simulink model "window"  (R2020a)
settings: Solver=VariableStepAuto  StartTime=0.0  StopTime=20000/f  RelTol=1e-3
InitFcn:
  | f = 256e6;
  | fs = 1.024e9;
  | delay = 0;
values from neighbouring files (symbols this model uses):
  fc_rx = 110e6    (= 110000000)    [spectrum_analyzer_setup.m]
  fc_tx = 110e6    (= 110000000)    [spectrum_analyzer_setup.m]
  SymbolRate = 1e6    (= 1000000)    [spectrum_analyzer_setup.m]
undefined symbols (not defined in the file or in its folder): designMultirateFIR, F_CICI, F_RRC, firhalfband
libraries: hdlsllib x14, dspmlti4 x6, dspfdesign x4, dspsrcs4 x3, simulink x2, dsparch4 x2, commfilt2 x2, commrandsrc3 x1, commdigbbndpm3 x1
settings Model: SimulationMode=accelerator  Creator=ckb13136  LastModifiedBy=david
settings DataIOCC: ReturnWorkspaceOutputs=off
settings OptimizationCC: BlockReduction=off  ConditionallyExecuteInputs=off  DefaultParameterBehavior=Inlined
settings DebuggingCC: AlgebraicLoopMsg=error  ArithmeticOperatorsInVariantConditions=warning
settings HardwareCC: ProdBitPerPointer=32  ProdBitPerSizeT=32  ProdBitPerPtrDiffT=32  ProdLargestAtomicFloat=None  ProdIntDivRoundTo=Undefined  ProdEndianess=Unspecified  ProdWordSize=32  ProdHWDeviceType=ASIC/FPGA->ASIC/FPGA  TargetBitPerPointer=64  TargetBitPerSizeT=64  TargetBitPerPtrDiffT=64  TargetLongLongMode=on  TargetIntDivRoundTo=Zero  TargetEndianess=LittleEndian  TargetWordSize=64  TargetHWDeviceType=Custom Processor->MATLAB Host Computer  ProdEqTarget=off
settings SFSimCC: SimUseLocalCustomCode=off  CustomCodeUndefinedFunction=UseInterfaceOnly
settings RTWCC: RTWUseLocalCustomCode=off

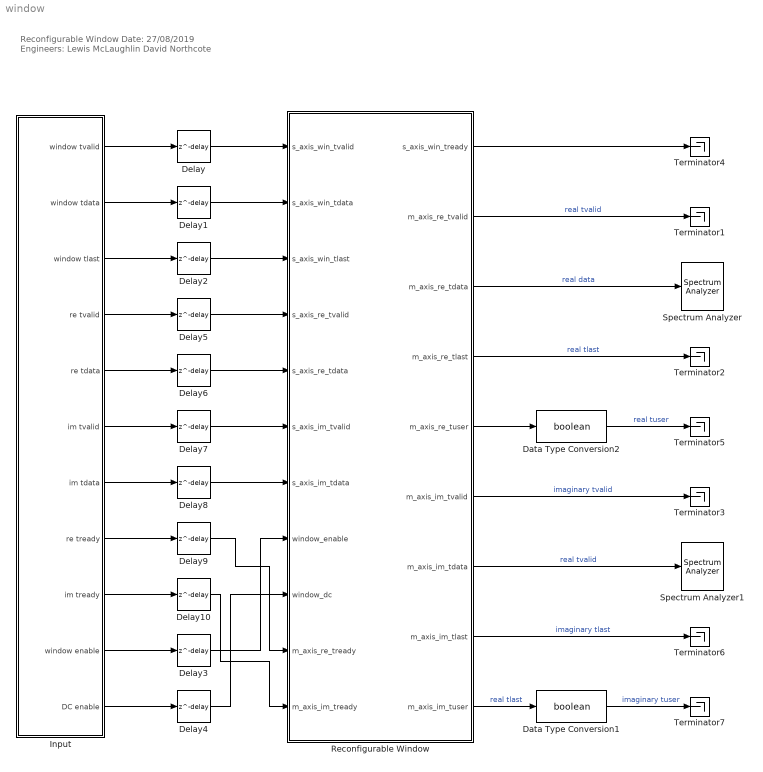
== system window ==
  note: Reconfigurable Window
      | Date: 27/08/2019
      | Engineers: Lewis McLaughlin
      | David Northcote
  Data Type Conversion1 : DataTypeConversion  OutDataTypeStr=boolean
  Data Type Conversion2 : DataTypeConversion  OutDataTypeStr=boolean
  Delay{,1..10} (11 alike) : Delay  DelayLength=delay
  Input : Subsystem  mask{window_length_mask=2048, window_type_mask=Debug, factor=1, f_hz=1e6, typeIn=Constant High, amplitude=0.990, DC=0.0, win_en=on, DC_en=off}
      mask prompts: window_length_mask "Window Length:"; window_type_mask "Window Type:"; factor "Downsample Factor:"; f_hz "Sine Frequency (Hz):"; typeIn "Input Type:"; DC "DC Component"; win_en "Window"; DC_en "DC Block"
      mask init:
      | % Parameters
      | if strcmpi(get_param(gcb, 'window_type_mask'), 'Hamming')
      |     window_type = 0;
      | elseif strcmpi(get_param(gcb, 'window_type_mask'), 'Hann')
      |     window_type = 1;
      | elseif strcmpi(get_param(gcb, 'window_type_mask'), 'Blackman')
      |     window_type = 2;
      | elseif strcmpi(get_param(gcb, 'window_type_mask'), 'Rectangular')
      |     window_type = 3;
      | elseif strcmpi(get_param(gcb, 'window_type_mask'), 'Debug')
      |     window_type = 4;
      | end
      | 
      | window_length = str2num(get_param(gcb, 'window_length_mask'));
      | 
      | % Input
      | if strcmpi(get_param(gcb,'typeIn'),'Constant High')
      |     input_type = 0;
      | elseif strcmpi(get_param(gcb,'typeIn'),'Sine Wave')
      |     input_type = 1;
      | elseif strcmpi(get_param(gcb,'typeIn'),'RF')
      |     input_type = 2;
      | end
      mask TypeOptions window_type_mask: Hamming | Hann | Blackman | Rectangular | Debug
      mask TypeOptions typeIn: Sine Wave | Constant High | RF
      mask DialogControl DescGroupVar Prompt: Input to Window Block
      mask DialogControl DescTextVar Prompt: Update the window parameters and input type as the system runs. A constant high input allows for the window shape to be observed with respect to time.
      mask DialogControl InputGroupVar Prompt: Input
      mask DialogControl EnableGroupVat Prompt: Enable
  Reconfigurable Window : Subsystem  AncestorBlock=lib_window/Reconfigurable Window  TreatAsAtomicUnit=on  VariantControl=Variant  mask{window_size=2048}
      mask prompts: window_size "Maximum Window Length:"
      mask DialogControl DescGroupVar Prompt: AXI-Stream Window
      mask DialogControl DescTextVar Prompt: When changing the window size, ensure the FIFOs under this mask are at least double maximum window size. Window size should be a power of two.
  Spectrum Analyzer : SpectrumAnalyzer
  Spectrum Analyzer1 : SpectrumAnalyzer
  Terminator{1..7} (7 alike) : Terminator
  wires:
  Input/4(re tvalid) -> Delay5/1
  Input/3(window tlast) -> Delay2/1
  Input/1(window tvalid) -> Delay/1
  Input/5(re tdata) -> Delay6/1
  Input/2(window tdata) -> Delay1/1
  Input/6(im tvalid) -> Delay7/1
  Input/7(im tdata) -> Delay8/1
  Input/9(im tready) -> Delay10/1
  Input/8(re tready) -> Delay9/1
  Delay10/1 -> Reconfigurable Window/11(m_axis_im_tready)
  Delay2/1 -> Reconfigurable Window/3(s_axis_win_tlast)
  Input/10(window enable) -> Delay3/1
  Delay5/1 -> Reconfigurable Window/4(s_axis_re_tvalid)
  Delay7/1 -> Reconfigurable Window/6(s_axis_im_tvalid)
  Delay9/1 -> Reconfigurable Window/10(m_axis_re_tready)
  Delay6/1 -> Reconfigurable Window/5(s_axis_re_tdata)
  Delay8/1 -> Reconfigurable Window/7(s_axis_im_tdata)
  Delay1/1 -> Reconfigurable Window/2(s_axis_win_tdata)
  Delay/1 -> Reconfigurable Window/1(s_axis_win_tvalid)
  Input/11(DC enable) -> Delay4/1
  Delay3/1 -> Reconfigurable Window/8(window_enable)
  Delay4/1 -> Reconfigurable Window/9(window_dc)
  Reconfigurable Window/4(m_axis_re_tlast) -> Terminator2/1  "real tlast"
  Reconfigurable Window/7(m_axis_im_tdata) -> Spectrum Analyzer1/1  "real tvalid"
  Reconfigurable Window/3(m_axis_re_tdata) -> Spectrum Analyzer/1  "real data"
  Reconfigurable Window/1(s_axis_win_tready) -> Terminator4/1
  Reconfigurable Window/2(m_axis_re_tvalid) -> Terminator1/1  "real tvalid"
  Reconfigurable Window/5(m_axis_re_tuser) -> Data Type Conversion2/1
  Reconfigurable Window/6(m_axis_im_tvalid) -> Terminator3/1  "imaginary tvalid"
  Reconfigurable Window/8(m_axis_im_tlast) -> Terminator6/1  "imaginary tlast"
  Data Type Conversion2/1 -> Terminator5/1  "real tuser"
  Reconfigurable Window/9(m_axis_im_tuser) -> Data Type Conversion1/1  "real tlast"
  Data Type Conversion1/1 -> Terminator7/1  "imaginary tuser"

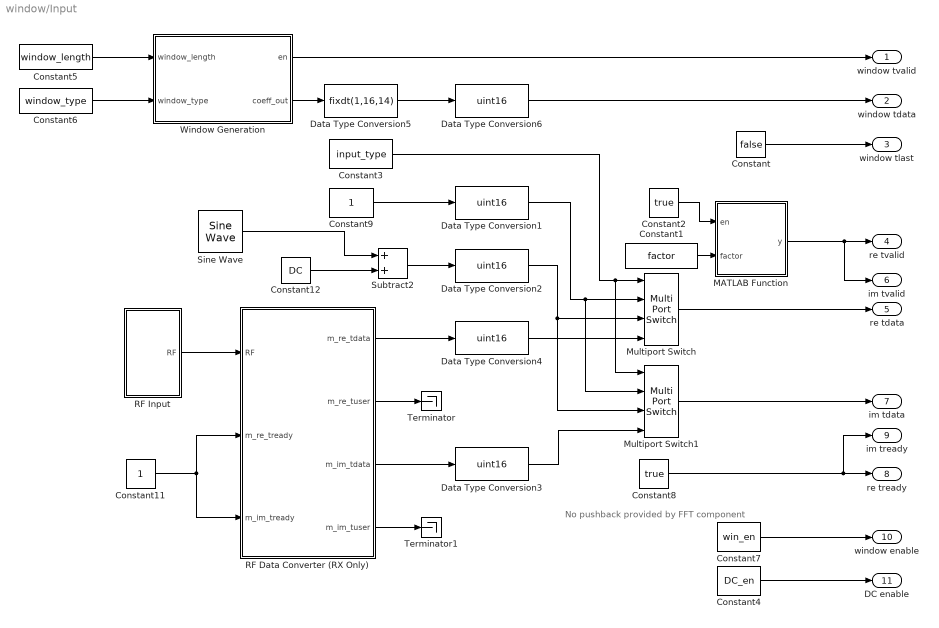
== system window/Input ==
  note: No pushback provided by FFT component
  Constant : Constant  Value=false  VectorParams1D=off  OutDataTypeStr=boolean  SampleTime=1/f
  Constant1 : Constant  Value=factor  SampleTime=1/f
  Constant11 : Constant  SampleTime=1/f
  Constant12 : Constant  Value=DC  VectorParams1D=off  OutDataTypeStr=fixdt(1,16,15)  SampleTime=1/f
  Constant2 : Constant  Value=true  SampleTime=1/f
  Constant3 : Constant  Value=input_type  SampleTime=1/f
  Constant4 : Constant  Value=DC_en  OutDataTypeStr=boolean  SampleTime=1/f
  Constant5 : Constant  Value=window_length  SampleTime=1/f
  Constant6 : Constant  Value=window_type  SampleTime=1/f
  Constant7 : Constant  Value=win_en  OutDataTypeStr=boolean  SampleTime=1/f
  Constant8 : Constant  Value=true  SampleTime=1/f
  Constant9 : Constant  OutDataTypeStr=fixdt(1,16,15)  SampleTime=1/f
  Data Type Conversion1 : DataTypeConversion  OutDataTypeStr=uint16  ConvertRealWorld=Stored Integer (SI)
  Data Type Conversion2 : DataTypeConversion  OutDataTypeStr=uint16  ConvertRealWorld=Stored Integer (SI)
  Data Type Conversion3 : DataTypeConversion  OutDataTypeStr=uint16
  Data Type Conversion4 : DataTypeConversion  OutDataTypeStr=uint16
  Data Type Conversion5 : DataTypeConversion  OutDataTypeStr=fixdt(1,16,14)
  Data Type Conversion6 : DataTypeConversion  OutDataTypeStr=uint16  ConvertRealWorld=Stored Integer (SI)
  MATLAB Function : MATLAB Function  TreatAsAtomicUnit=on
  Multiport Switch : MultiPortSwitch  DataPortOrder=Zero-based contiguous  zeroidx=on
  Multiport Switch1 : MultiPortSwitch  DataPortOrder=Zero-based contiguous  zeroidx=on
  RF Data Converter (RX Only) : Subsystem
  RF Input : Subsystem
  Sine Wave : dspsrcs4/Sine Wave  Amplitude=amplitude  Frequency=f_hz  Phase=0  SampleMode=Discrete  OutComplex=Real  CompMethod=Table lookup  TableSize=Speed  SampleTime=1/f  SamplesPerFrame=1  ResetState=Restart at time zero  OutputFrames=off  dataType=Fixed-point  wordLen=16  udDataType=sfix(16)  fracBitsMode=User-defined  numFracBits=15  OutDataTypeStr=fixdt(1,16,15)  LastOutDataTypeStr=fixdt(1,16,15)
  Subtract2 : Sum
  Terminator : Terminator
  Terminator1 : Terminator
  Window Generation : MATLAB Function  TreatAsAtomicUnit=on
  window tvalid : Outport  VectorParamsAs1DForOutWhenUnconnected=off
  window tdata : Outport  Port=2  VectorParamsAs1DForOutWhenUnconnected=off
  window tlast : Outport  Port=3  VectorParamsAs1DForOutWhenUnconnected=off
  re tvalid : Outport  Port=4  VectorParamsAs1DForOutWhenUnconnected=off
  re tdata : Outport  Port=5  VectorParamsAs1DForOutWhenUnconnected=off
  im tvalid : Outport  Port=6  VectorParamsAs1DForOutWhenUnconnected=off
  im tdata : Outport  Port=7  VectorParamsAs1DForOutWhenUnconnected=off
  re tready : Outport  Port=8  VectorParamsAs1DForOutWhenUnconnected=off
  im tready : Outport  Port=9  VectorParamsAs1DForOutWhenUnconnected=off
  window enable : Outport  Port=10  VectorParamsAs1DForOutWhenUnconnected=off
  DC enable : Outport  Port=11  VectorParamsAs1DForOutWhenUnconnected=off
  wires:
  Window Generation/2(coeff_out) -> Data Type Conversion5/1
  Constant9/1 -> Data Type Conversion1/1
  Constant3/1 -> Multiport Switch1/1, Multiport Switch/1
  Constant5/1 -> Window Generation/1(window_length)
  Constant6/1 -> Window Generation/2(window_type)
  RF Input/1(RF) -> RF Data Converter (RX Only)/1(RF)
  RF Data Converter (RX Only)/1(m_re_tdata) -> Data Type Conversion4/1
  Constant11/1 -> RF Data Converter (RX Only)/2(m_re_tready), RF Data Converter (RX Only)/3(m_im_tready)
  RF Data Converter (RX Only)/2(m_re_tuser) -> Terminator/1
  RF Data Converter (RX Only)/4(m_im_tuser) -> Terminator1/1
  RF Data Converter (RX Only)/3(m_im_tdata) -> Data Type Conversion3/1
  Data Type Conversion3/1 -> Multiport Switch1/4
  Data Type Conversion4/1 -> Multiport Switch/4
  Subtract2/1 -> Data Type Conversion2/1
  Data Type Conversion1/1 -> Multiport Switch1/2, Multiport Switch/2
  Data Type Conversion5/1 -> Data Type Conversion6/1
  Sine Wave/1 -> Subtract2/1
  Constant12/1 -> Subtract2/2
  Data Type Conversion2/1 -> Multiport Switch1/3, Multiport Switch/3
  Window Generation/1(en) -> window tvalid/1
  Data Type Conversion6/1 -> window tdata/1
  MATLAB Function/1(y) -> im tvalid/1, re tvalid/1
  Constant/1 -> window tlast/1
  Multiport Switch/1 -> re tdata/1
  Constant8/1 -> im tready/1, re tready/1
  Multiport Switch1/1 -> im tdata/1
  Constant2/1 -> MATLAB Function/1(en)
  Constant1/1 -> MATLAB Function/2(factor)
  Constant7/1 -> window enable/1
  Constant4/1 -> DC enable/1

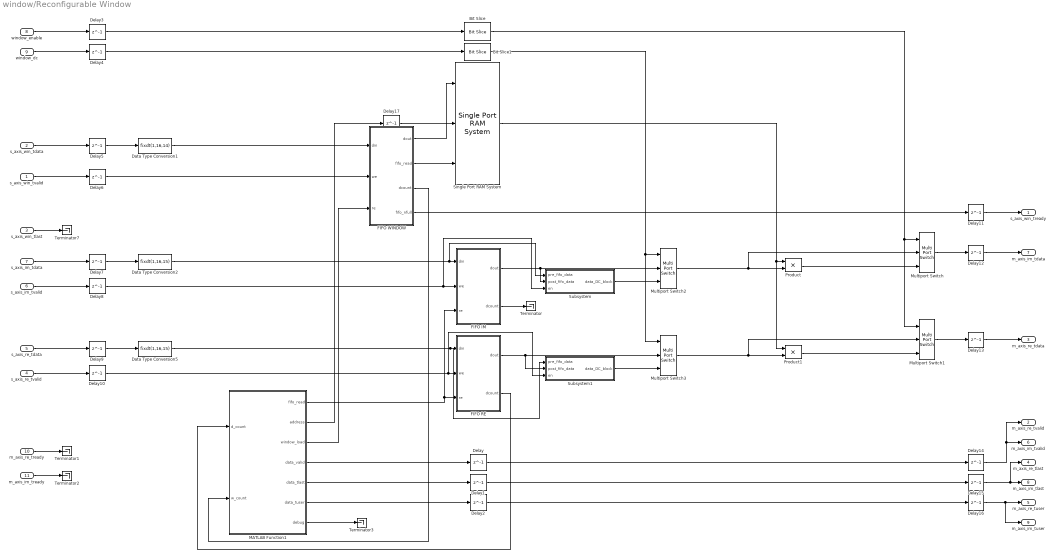
== system window/Reconfigurable Window ==
  s_axis_win_tvalid : Inport
  s_axis_win_tdata : Inport  Port=2
  s_axis_win_tlast : Inport  Port=3
  s_axis_re_tvalid : Inport  Port=4
  s_axis_re_tdata : Inport  Port=5
  s_axis_im_tvalid : Inport  Port=6
  s_axis_im_tdata : Inport  Port=7
  window_enable : Inport  Port=8
  window_dc : Inport  Port=9
  m_axis_re_tready : Inport  Port=10
  m_axis_im_tready : Inport  Port=11
  Bit Slice : hdlsllib/Logic and Bit Operations/Bit Slice  lidx=0  ridx=0
      settings: SourceProductBaseCode=SL
  Bit Slice1 : hdlsllib/Logic and Bit Operations/Bit Slice  lidx=0  ridx=0
      settings: SourceProductBaseCode=SL
  Data Type Conversion1 : DataTypeConversion  OutDataTypeStr=fixdt(1,16,14)  ConvertRealWorld=Stored Integer (SI)
  Data Type Conversion2 : DataTypeConversion  OutDataTypeStr=fixdt(1,16,15)  ConvertRealWorld=Stored Integer (SI)
  Data Type Conversion5 : DataTypeConversion  OutDataTypeStr=fixdt(1,16,15)  ConvertRealWorld=Stored Integer (SI)
  Delay{,1..17} (18 alike) : Delay  DelayLength=1
  FIFO IM : Subsystem
  FIFO RE : Subsystem
  FIFO WINDOW : Subsystem
  MATLAB Function1 : MATLAB Function  TreatAsAtomicUnit=on
  Multiport Switch{,1..3} (4 alike) : MultiPortSwitch  DataPortOrder=Zero-based contiguous  Inputs=2  zeroidx=on
  Product : Product  OutDataTypeStr=fixdt(1,16,15)  SaturateOnIntegerOverflow=on
  Product1 : Product  OutDataTypeStr=fixdt(1,16,15)  SaturateOnIntegerOverflow=on
  Single Port RAM System : hdlsllib/HDL RAMs/Single Port RAM System  RAMType=Single port  WriteOutputValue=New data  RAMInitialValue=0  SimulateUsing=Code generation
      settings: SourceProductBaseCode=SL
  Subsystem : Subsystem
  Subsystem1 : Subsystem
  Terminator{,1..3,7} (5 alike) : Terminator
  s_axis_win_tready : Outport  VectorParamsAs1DForOutWhenUnconnected=off
  m_axis_re_tvalid : Outport  Port=2  VectorParamsAs1DForOutWhenUnconnected=off
  m_axis_re_tdata : Outport  Port=3  VectorParamsAs1DForOutWhenUnconnected=off
  m_axis_re_tlast : Outport  Port=4  VectorParamsAs1DForOutWhenUnconnected=off
  m_axis_re_tuser : Outport  Port=5  VectorParamsAs1DForOutWhenUnconnected=off
  m_axis_im_tvalid : Outport  Port=6  VectorParamsAs1DForOutWhenUnconnected=off
  m_axis_im_tdata : Outport  Port=7  VectorParamsAs1DForOutWhenUnconnected=off
  m_axis_im_tlast : Outport  Port=8  VectorParamsAs1DForOutWhenUnconnected=off
  m_axis_im_tuser : Outport  Port=9  VectorParamsAs1DForOutWhenUnconnected=off
  wires:
  FIFO RE/1(dout) -> Multiport Switch3/2, Subsystem1/2(post_fifo_data)
  Data Type Conversion5/1 -> FIFO RE/1(din), Subsystem1/1(pre_fifo_data)
  Data Type Conversion2/1 -> FIFO IM/1(din), Subsystem/1(pre_fifo_data)
  Data Type Conversion1/1 -> FIFO WINDOW/1(din)
  FIFO WINDOW/1(dout) -> Single Port RAM System/1
  MATLAB Function1/2(address) -> Delay17/1
  MATLAB Function1/3(window_load) -> FIFO WINDOW/3(re)
  s_axis_win_tdata/1 -> Delay5/1
  s_axis_win_tvalid/1 -> Delay6/1
  FIFO WINDOW/3(dcount) -> MATLAB Function1/2(w_count)
  FIFO RE/2(dcount) -> MATLAB Function1/1(d_count)
  s_axis_im_tdata/1 -> Delay7/1
  s_axis_im_tvalid/1 -> Delay8/1
  s_axis_re_tdata/1 -> Delay9/1
  s_axis_re_tvalid/1 -> Delay10/1
  MATLAB Function1/1(fifo_read) -> FIFO RE/3(re), FIFO IM/3(re)
  Subsystem1/1(data_DC_block) -> Multiport Switch3/3
  Subsystem/1(data_DC_block) -> Multiport Switch2/3
  Product1/1 -> Multiport Switch1/3
  Product/1 -> Multiport Switch/3
  Single Port RAM System/1 -> Product1/1, Product/1
  FIFO IM/2(dcount) -> Terminator/1
  Bit Slice1/1 -> Multiport Switch3/1, Multiport Switch2/1
  Bit Slice/1 -> Multiport Switch1/1, Multiport Switch/1
  MATLAB Function1/6(data_tuser) -> Delay2/1
  MATLAB Function1/5(data_tlast) -> Delay1/1
  MATLAB Function1/4(data_valid) -> Delay/1
  s_axis_win_tlast/1 -> Terminator7/1
  FIFO WINDOW/2(fifo_read) -> Single Port RAM System/3
  FIFO WINDOW/4(fifo_nfull) -> Delay11/1
  Multiport Switch1/1 -> Delay13/1
  Multiport Switch/1 -> Delay12/1
  m_axis_re_tready/1 -> Terminator1/1
  m_axis_im_tready/1 -> Terminator2/1
  Delay/1 -> Delay14/1
  Delay1/1 -> Delay15/1
  Delay2/1 -> Delay16/1
  window_enable/1 -> Delay3/1
  Multiport Switch2/1 -> Multiport Switch/2, Product/2
  Multiport Switch3/1 -> Multiport Switch1/2, Product1/2
  FIFO IM/1(dout) -> Subsystem/2(post_fifo_data), Multiport Switch2/2
  window_dc/1 -> Delay4/1
  Delay3/1 -> Bit Slice/1
  Delay4/1 -> Bit Slice1/1
  Delay5/1 -> Data Type Conversion1/1
  Delay6/1 -> FIFO WINDOW/2(we)
  Delay7/1 -> Data Type Conversion2/1
  Delay8/1 -> FIFO IM/2(we), Subsystem/3(en)
  Delay9/1 -> Data Type Conversion5/1
  Delay10/1 -> FIFO RE/2(we), Subsystem1/3(en)
  Delay11/1 -> s_axis_win_tready/1
  Delay12/1 -> m_axis_im_tdata/1
  Delay13/1 -> m_axis_re_tdata/1
  Delay14/1 -> m_axis_re_tvalid/1, m_axis_im_tvalid/1
  Delay15/1 -> m_axis_im_tlast/1, m_axis_re_tlast/1
  Delay16/1 -> m_axis_re_tuser/1, m_axis_im_tuser/1
  Delay17/1 -> Single Port RAM System/2
  MATLAB Function1/7(debug) -> Terminator3/1

== system window/Input/RF Data Converter (RX Only) ==
  RF : Inport
  m_re_tready : Inport  Port=2
  m_im_tready : Inport  Port=3
  Complex To AXI-Stream : Subsystem
  RF Data Converter Rx : Subsystem
  m_re_tdata : Outport  VectorParamsAs1DForOutWhenUnconnected=off
  m_re_tuser : Outport  Port=2  VectorParamsAs1DForOutWhenUnconnected=off
  m_im_tdata : Outport  Port=3  VectorParamsAs1DForOutWhenUnconnected=off
  m_im_tuser : Outport  Port=4  VectorParamsAs1DForOutWhenUnconnected=off
  wires:
  Complex To AXI-Stream/3(m_im_tdata) -> m_im_tdata/1
  RF/1 -> RF Data Converter Rx/1(Rx)
  Complex To AXI-Stream/1(m_re_tdata) -> m_re_tdata/1
  m_im_tready/1 -> Complex To AXI-Stream/4(m_im_tready)
  RF Data Converter Rx/2(Q_out) -> Complex To AXI-Stream/2(im_data)
  m_re_tready/1 -> Complex To AXI-Stream/3(m_re_tready)
  RF Data Converter Rx/1(I_out) -> Complex To AXI-Stream/1(re_data)
  Complex To AXI-Stream/2(m_re_tuser) -> m_re_tuser/1
  Complex To AXI-Stream/4(m_im_tuser) -> m_im_tuser/1

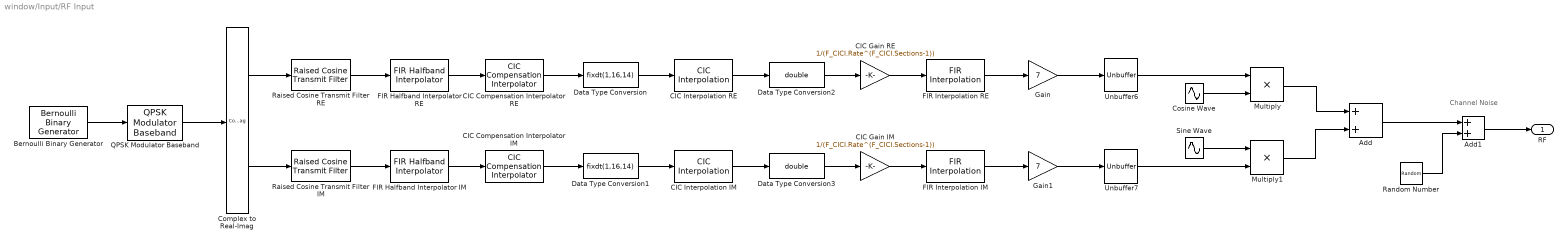
== system window/Input/RF Input ==
  note: Channel Noise
  Add : Sum
  Add1 : Sum
  Bernoulli Binary Generator : commrandsrc3/Bernoulli Binary Generator  ProbabilityOfZero=0.5  SeedSource=Parameter  Seed=0  SampleTime=1/(SymbolRate*2)  SamplesPerFrame=2  OutputDataType=double  SimulateUsing=Interpreted execution
  CIC Interpolation IM : dspmlti4/CIC Interpolation  filtFrom=Dialog parameters  filtobj=CICINTERP  ftype=Interpolator  R=F_CICI.Rate  M=F_CICI.DifferentialDelay  N=F_CICI.Sections  filterInternals=Full precision  BPS=[16 16 16 16]  FLPS=0  outputWordLength=32  outputFracLength=0  launchFVT=off  InputProcessing=Columns as channels (frame based)  framing=Enforce single-rate processing  OutputFrames=off
      settings: SourceProductBaseCode=DS
  CIC Interpolation RE : dspmlti4/CIC Interpolation  filtFrom=Dialog parameters  filtobj=CICINTERP  ftype=Interpolator  R=F_CICI.Rate  M=F_CICI.DifferentialDelay  N=F_CICI.Sections  filterInternals=Full precision  BPS=[16 16 16 16]  FLPS=0  outputWordLength=32  outputFracLength=0  launchFVT=off  InputProcessing=Columns as channels (frame based)  framing=Enforce single-rate processing  OutputFrames=off
      settings: SourceProductBaseCode=DS
  CIC Compensation Interpolator IM : dspfdesign/CIC Compensation Interpolator  CICRateChangeFactor=F_CICI.Rate  CICNumSections=F_CICI.Sections  CICDifferentialDelay=F_CICI.DifferentialDelay  InterpolationFactor=F_CICC.Rate  DesignForMinimumOrder=on  FilterOrder=12  PassbandFrequency=F_CICC.Passband  StopbandFrequency=F_CICC.Stopband  PassbandRipple=F_CICC.Ripple  StopbandAttenuation=F_CICC.StopbandAttenuation  InheritSampleRate=off  SampleRate=F_CICC.SampleRate  SimulateUsing=Code generation  roundingMode=Floor  coeffsDataTypeStr=fixdt(1,16)
      settings: SourceProductBaseCode=DS
  CIC Compensation Interpolator RE : dspfdesign/CIC Compensation Interpolator  CICRateChangeFactor=F_CICI.Rate  CICNumSections=F_CICI.Sections  CICDifferentialDelay=F_CICI.DifferentialDelay  InterpolationFactor=F_CICC.Rate  DesignForMinimumOrder=on  FilterOrder=12  PassbandFrequency=F_CICC.Passband  StopbandFrequency=F_CICC.Stopband  PassbandRipple=F_CICC.Ripple  StopbandAttenuation=F_CICC.StopbandAttenuation  InheritSampleRate=off  SampleRate=F_CICC.SampleRate  SimulateUsing=Code generation  roundingMode=Floor  coeffsDataTypeStr=fixdt(1,16)
      settings: SourceProductBaseCode=DS
  CIC Gain IM : Gain  Gain=1/(F_CICI.Rate^(F_CICI.Sections-1))
  CIC Gain RE : Gain  Gain=1/(F_CICI.Rate^(F_CICI.Sections-1))
  Complex to Real-Imag : ComplexToRealImag
  Cosine Wave : Sin  Frequency=2*pi*fc_tx  Phase=pi/2  SampleTime=0
  Data Type Conversion : DataTypeConversion  OutDataTypeStr=fixdt(1,16,14)
  Data Type Conversion1 : DataTypeConversion  OutDataTypeStr=fixdt(1,16,14)
  Data Type Conversion2 : DataTypeConversion  OutDataTypeStr=double
  Data Type Conversion3 : DataTypeConversion  OutDataTypeStr=double
  FIR Interpolation IM : dspmlti4/FIR Interpolation  FilterSource=Auto  PrivateCoeffs=0  h=designMultirateFIR(3,1)  L=8  FilterObject=FINTERP  InputProcessing=Columns as channels (frame based)  framing=Enforce single-rate processing  outputBufInitCond=0  roundingMode=Floor  overflowMode=off  firstCoeffDataTypeStr=Inherit: Same word length as input  firstCoeffMin=[]  firstCoeffMax=[]  firstCoeffLastDataTypeStr=Inherit: Same word length as input  outputDataTypeStr=Inherit: Same as accumulator  outputMin=[]  outputMax=[]  outputLastDataTypeStr=Inherit: Same as accumulator
  FIR Interpolation RE : dspmlti4/FIR Interpolation  FilterSource=Auto  PrivateCoeffs=0  h=designMultirateFIR(3,1)  L=8  FilterObject=FINTERP  InputProcessing=Columns as channels (frame based)  framing=Enforce single-rate processing  outputBufInitCond=0  roundingMode=Floor  overflowMode=off  firstCoeffDataTypeStr=Inherit: Same word length as input  firstCoeffMin=[]  firstCoeffMax=[]  firstCoeffLastDataTypeStr=Inherit: Same word length as input  outputDataTypeStr=Inherit: Same as accumulator  outputMin=[]  outputMax=[]  outputLastDataTypeStr=Inherit: Same as accumulator
  FIR Halfband Interpolator IM : dspfdesign/FIR Halfband Interpolator  Specification=Transition width and stopband attenuation  FilterOrder=52  TransitionWidth=F_HB.TransitionWidth  StopbandAttenuation=F_HB.StopbandAttenuation  Numerator=2*firhalfband( 'minorder', 0.407, 1e-4 )  FilterBankInputPort=off  InheritSampleRate=off  SampleRate=F_HB.SampleRate  SimulateUsing=Code generation  roundingMode=Floor  coeffsDataTypeStr=fixdt(1,16)
      settings: SourceProductBaseCode=DS
  FIR Halfband Interpolator RE : dspfdesign/FIR Halfband Interpolator  Specification=Transition width and stopband attenuation  FilterOrder=52  TransitionWidth=F_HB.TransitionWidth  StopbandAttenuation=F_HB.StopbandAttenuation  Numerator=2*firhalfband( 'minorder', 0.407, 1e-4 )  FilterBankInputPort=off  InheritSampleRate=off  SampleRate=F_HB.SampleRate  SimulateUsing=Code generation  roundingMode=Floor  coeffsDataTypeStr=fixdt(1,16)
      settings: SourceProductBaseCode=DS
  Gain : Gain  Gain=7
  Gain1 : Gain  Gain=7
  Multiply : Product
  Multiply1 : Product
  QPSK Modulator Baseband : commdigbbndpm3/QPSK Modulator Baseband  InType=Bit  Enc=Gray  Ph=pi/4  outDtype=double  outWordLen=16  outUDDataType=sfix(16)  outFracLenMode=Best precision  outFracLen=15  outDataTypeStr=double  outLastDataTypeStr=double
  Raised Cosine Transmit Filter IM : commfilt2/Raised Cosine Transmit Filter  filtType=Square root  R=F_RRC.RollOff  filtSpan=F_RRC.FilterSpan  N=F_RRC.Rate  filterGain=F_RRC.LinearGain  InputProcessing=Columns as channels (frame based)  RateOptions=Allow multirate processing  framing=Mute  checkCoeff=off  variableName=rcTxFilt1  checkGain=Normalized  sampMode=Mute  saveAsFlag=0  currentFiltSpan=10  D=(10)/2  launchFVT=on  roundingMode=Floor  overflowMode=off  coeffDataTypeStr=Inherit: Same word length as input  coeffMin=[]  coeffMax=[]  coeffLastDataTypeStr=Inherit: Same word length as input  outputDataTypeStr=Inherit: Same as accumulator  outputMin=[]  outputMax=[]  outputLastDataTypeStr=Inherit: Same as accumulator
  Raised Cosine Transmit Filter RE : commfilt2/Raised Cosine Transmit Filter  filtType=Square root  R=F_RRC.RollOff  filtSpan=F_RRC.FilterSpan  N=F_RRC.Rate  filterGain=F_RRC.LinearGain  InputProcessing=Columns as channels (frame based)  RateOptions=Allow multirate processing  framing=Mute  checkCoeff=off  variableName=rcTxFilt  checkGain=Normalized  sampMode=Mute  saveAsFlag=0  currentFiltSpan=10  D=(10)/2  launchFVT=on  roundingMode=Floor  overflowMode=off  coeffDataTypeStr=Inherit: Same word length as input  coeffMin=[]  coeffMax=[]  coeffLastDataTypeStr=Inherit: Same word length as input  outputDataTypeStr=Inherit: Same as accumulator  outputMin=[]  outputMax=[]  outputLastDataTypeStr=Inherit: Same as accumulator
  Random Number : RandomNumber  Variance=0.05  SampleTime=1/fs
  Sine Wave : Sin  Frequency=2*pi*fc_tx  SampleTime=0
  Unbuffer6 : Unbuffer
  Unbuffer7 : Unbuffer
  RF : Outport  VectorParamsAs1DForOutWhenUnconnected=off
  wires:
  Gain1/1 -> Unbuffer7/1
  Gain/1 -> Unbuffer6/1
  Unbuffer7/1 -> Multiply1/2
  Unbuffer6/1 -> Multiply/1
  Random Number/1 -> Add1/2
  Add1/1 -> RF/1
  Add/1 -> Add1/1
  FIR Interpolation IM/1 -> Gain1/1
  Sine Wave/1 -> Multiply1/1
  Cosine Wave/1 -> Multiply/2
  FIR Interpolation RE/1 -> Gain/1
  Multiply1/1 -> Add/2
  Multiply/1 -> Add/1
  CIC Gain IM/1 -> FIR Interpolation IM/1
  CIC Gain RE/1 -> FIR Interpolation RE/1
  CIC Interpolation IM/1 -> Data Type Conversion3/1
  Data Type Conversion3/1 -> CIC Gain IM/1
  Data Type Conversion2/1 -> CIC Gain RE/1
  Data Type Conversion1/1 -> CIC Interpolation IM/1
  Data Type Conversion/1 -> CIC Interpolation RE/1
  CIC Interpolation RE/1 -> Data Type Conversion2/1
  CIC Compensation Interpolator IM/1 -> Data Type Conversion1/1
  CIC Compensation Interpolator RE/1 -> Data Type Conversion/1
  FIR Halfband Interpolator IM/1 -> CIC Compensation Interpolator IM/1
  FIR Halfband Interpolator RE/1 -> CIC Compensation Interpolator RE/1
  Raised Cosine Transmit Filter IM/1 -> FIR Halfband Interpolator IM/1
  Raised Cosine Transmit Filter RE/1 -> FIR Halfband Interpolator RE/1
  Complex to Real-Imag/2 -> Raised Cosine Transmit Filter IM/1
  QPSK Modulator Baseband/1 -> Complex to Real-Imag/1
  Complex to Real-Imag/1 -> Raised Cosine Transmit Filter RE/1
  Bernoulli Binary Generator/1 -> QPSK Modulator Baseband/1

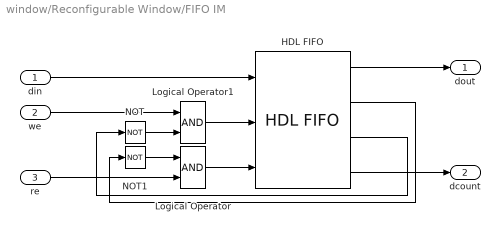
== system window/Reconfigurable Window/FIFO IM ==
  din : Inport
  we : Inport  Port=2
  re : Inport  Port=3
  HDL FIFO : hdlsllib/HDL RAMs/HDL FIFO  fifo_size=2*window_size  mode=Classic  ratio=1  push_msg=Warning  pop_msg=Warning  show_empty=on  show_full=on  show_num=on  LabelModeActiveChoice_Mode=Classic
      settings: SourceProductBaseCode=SL
  Logical Operator : Logic  AllPortsSameDT=off  OutDataTypeStr=boolean
  Logical Operator1 : Logic  AllPortsSameDT=off  OutDataTypeStr=boolean
  NOT : Logic  Operator=NOT  AllPortsSameDT=off  OutDataTypeStr=boolean
  NOT1 : Logic  Operator=NOT  AllPortsSameDT=off  OutDataTypeStr=boolean
  dout : Outport  VectorParamsAs1DForOutWhenUnconnected=off
  dcount : Outport  Port=2  VectorParamsAs1DForOutWhenUnconnected=off
  wires:
  Logical Operator/1 -> HDL FIFO/3
  Logical Operator1/1 -> HDL FIFO/2
  NOT/1 -> Logical Operator1/2
  NOT1/1 -> Logical Operator/1
  HDL FIFO/2 -> NOT1/1
  HDL FIFO/1 -> dout/1
  re/1 -> Logical Operator/2
  HDL FIFO/3 -> NOT/1
  we/1 -> Logical Operator1/1
  din/1 -> HDL FIFO/1
  HDL FIFO/4 -> dcount/1

== system window/Reconfigurable Window/FIFO RE ==
  din : Inport
  we : Inport  Port=2
  re : Inport  Port=3
  HDL FIFO : hdlsllib/HDL RAMs/HDL FIFO  fifo_size=2*window_size  mode=Classic  ratio=1  push_msg=Warning  pop_msg=Warning  show_empty=on  show_full=on  show_num=on  LabelModeActiveChoice_Mode=Classic
      settings: SourceProductBaseCode=SL
  Logical Operator : Logic  AllPortsSameDT=off  OutDataTypeStr=boolean
  Logical Operator1 : Logic  AllPortsSameDT=off  OutDataTypeStr=boolean
  NOT : Logic  Operator=NOT  AllPortsSameDT=off  OutDataTypeStr=boolean
  NOT1 : Logic  Operator=NOT  AllPortsSameDT=off  OutDataTypeStr=boolean
  dout : Outport  VectorParamsAs1DForOutWhenUnconnected=off
  dcount : Outport  Port=2  VectorParamsAs1DForOutWhenUnconnected=off
  wires:
  HDL FIFO/4 -> dcount/1
  din/1 -> HDL FIFO/1
  we/1 -> Logical Operator1/1
  HDL FIFO/3 -> NOT/1
  re/1 -> Logical Operator/2
  HDL FIFO/1 -> dout/1
  HDL FIFO/2 -> NOT1/1
  NOT1/1 -> Logical Operator/1
  NOT/1 -> Logical Operator1/2
  Logical Operator1/1 -> HDL FIFO/2
  Logical Operator/1 -> HDL FIFO/3

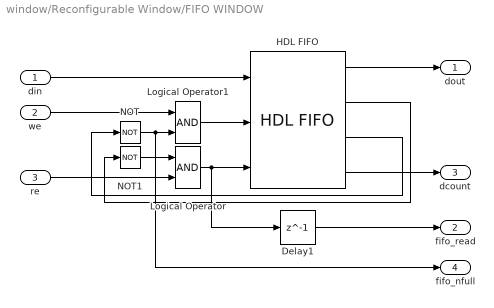
== system window/Reconfigurable Window/FIFO WINDOW ==
  din : Inport
  we : Inport  Port=2
  re : Inport  Port=3
  Delay1 : Delay  DelayLength=1
  HDL FIFO : hdlsllib/HDL RAMs/HDL FIFO  fifo_size=2*window_size  mode=Classic  ratio=1  push_msg=Warning  pop_msg=Warning  show_empty=on  show_full=on  show_num=on  LabelModeActiveChoice_Mode=Classic
      settings: SourceProductBaseCode=SL
  Logical Operator : Logic  AllPortsSameDT=off  OutDataTypeStr=boolean
  Logical Operator1 : Logic  AllPortsSameDT=off  OutDataTypeStr=boolean
  NOT : Logic  Operator=NOT  AllPortsSameDT=off  OutDataTypeStr=boolean
  NOT1 : Logic  Operator=NOT  AllPortsSameDT=off  OutDataTypeStr=boolean
  dout : Outport  VectorParamsAs1DForOutWhenUnconnected=off
  fifo_read : Outport  Port=2  VectorParamsAs1DForOutWhenUnconnected=off
  dcount : Outport  Port=3  VectorParamsAs1DForOutWhenUnconnected=off
  fifo_nfull : Outport  Port=4  VectorParamsAs1DForOutWhenUnconnected=off
  wires:
  Delay1/1 -> fifo_read/1
  HDL FIFO/4 -> dcount/1
  Logical Operator/1 -> HDL FIFO/3, Delay1/1
  HDL FIFO/2 -> NOT1/1
  HDL FIFO/1 -> dout/1
  Logical Operator1/1 -> HDL FIFO/2
  re/1 -> Logical Operator/2
  we/1 -> Logical Operator1/1
  HDL FIFO/3 -> NOT/1
  din/1 -> HDL FIFO/1
  NOT1/1 -> Logical Operator/1
  NOT/1 -> Logical Operator1/2, fifo_nfull/1

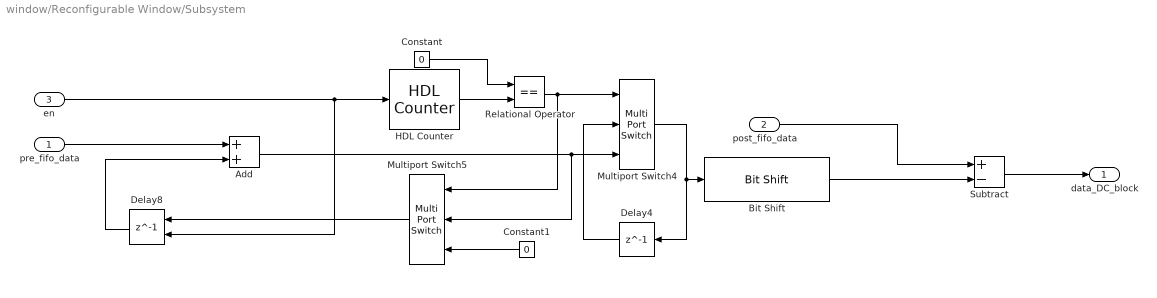
== system window/Reconfigurable Window/Subsystem ==
  pre_fifo_data : Inport
  post_fifo_data : Inport  Port=2
  en : Inport  Port=3
  Add : Sum  OutDataTypeStr=fixdt(1,32,15)
  Bit Shift : hdlsllib/Logic and Bit Operations/Bit Shift  mode=Shift Right Logical  N=log2(window_size)
  Constant : Constant  Value=0  OutDataTypeStr=fixdt(0,1,0)  SampleTime=1/f
  Constant1 : Constant  Value=0  OutDataTypeStr=fixdt(1,32,15)  SampleTime=1/f
  Delay4 : Delay  DelayLength=1
  Delay8 : Delay  DelayLength=1  ShowEnablePort=on
      settings: InputPortMap=u0,e6
  HDL Counter : hdlsllib/Sources/HDL Counter  CountType=Count limited  CountInit=1  CountStep=1  CountMax=window_size-1  CountFromType=Specify  CountFrom=0  CountResetPort=off  CountLoadPort=off  CountEnbPort=on  CountDirPort=off  CountDataType=Unsigned  CountWordLen=log2(window_size)  CountFracLen=0  CountSampTime=1
  Multiport Switch4 : MultiPortSwitch  DataPortOrder=Zero-based contiguous  Inputs=2  zeroidx=on
  Multiport Switch5 : MultiPortSwitch  DataPortOrder=Zero-based contiguous  Inputs=2  zeroidx=on
  Relational Operator : RelationalOperator  Operator===  OutDataTypeStr=boolean  RndMeth=Simplest
  Subtract : Sum  Inputs=+-  OutDataTypeStr=fixdt(1,16,15)
  data_DC_block : Outport
  wires:
  post_fifo_data/1 -> Subtract/1
  pre_fifo_data/1 -> Add/1
  Multiport Switch5/1 -> Delay8/1
  Bit Shift/1 -> Subtract/2
  Add/1 -> Multiport Switch4/3, Multiport Switch5/2
  Relational Operator/1 -> Multiport Switch5/1, Multiport Switch4/1
  Subtract/1 -> data_DC_block/1
  Constant/1 -> Relational Operator/1
  Multiport Switch4/1 -> Bit Shift/1, Delay4/1
  en/1 -> Delay8/2, HDL Counter/1
  Delay4/1 -> Multiport Switch4/2
  HDL Counter/1 -> Relational Operator/2
  Constant1/1 -> Multiport Switch5/3
  Delay8/1 -> Add/2

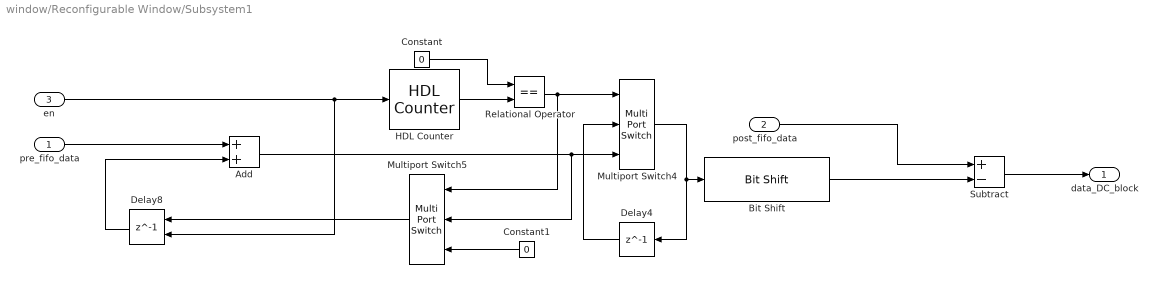
== system window/Reconfigurable Window/Subsystem1 ==
  pre_fifo_data : Inport
  post_fifo_data : Inport  Port=2
  en : Inport  Port=3
  Add : Sum  OutDataTypeStr=fixdt(1,32,15)
  Bit Shift : hdlsllib/Logic and Bit Operations/Bit Shift  mode=Shift Right Logical  N=log2(window_size)
  Constant : Constant  Value=0  OutDataTypeStr=fixdt(0,1,0)  SampleTime=1/f
  Constant1 : Constant  Value=0  OutDataTypeStr=fixdt(1,32,15)  SampleTime=1/f
  Delay4 : Delay  DelayLength=1
  Delay8 : Delay  DelayLength=1  ShowEnablePort=on
      settings: InputPortMap=u0,e6
  HDL Counter : hdlsllib/Sources/HDL Counter  CountType=Count limited  CountInit=1  CountStep=1  CountMax=window_size-1  CountFromType=Specify  CountFrom=0  CountResetPort=off  CountLoadPort=off  CountEnbPort=on  CountDirPort=off  CountDataType=Unsigned  CountWordLen=log2(window_size)  CountFracLen=0  CountSampTime=1
  Multiport Switch4 : MultiPortSwitch  DataPortOrder=Zero-based contiguous  Inputs=2  zeroidx=on
  Multiport Switch5 : MultiPortSwitch  DataPortOrder=Zero-based contiguous  Inputs=2  zeroidx=on
  Relational Operator : RelationalOperator  Operator===  OutDataTypeStr=boolean  RndMeth=Simplest
  Subtract : Sum  Inputs=+-  OutDataTypeStr=fixdt(1,16,15)
  data_DC_block : Outport
  wires:
  Delay8/1 -> Add/2
  Constant1/1 -> Multiport Switch5/3
  HDL Counter/1 -> Relational Operator/2
  Delay4/1 -> Multiport Switch4/2
  en/1 -> HDL Counter/1, Delay8/2
  Multiport Switch4/1 -> Delay4/1, Bit Shift/1
  Constant/1 -> Relational Operator/1
  Subtract/1 -> data_DC_block/1
  Relational Operator/1 -> Multiport Switch4/1, Multiport Switch5/1
  Add/1 -> Multiport Switch5/2, Multiport Switch4/3
  Bit Shift/1 -> Subtract/2
  Multiport Switch5/1 -> Delay8/1
  pre_fifo_data/1 -> Add/1
  post_fifo_data/1 -> Subtract/1

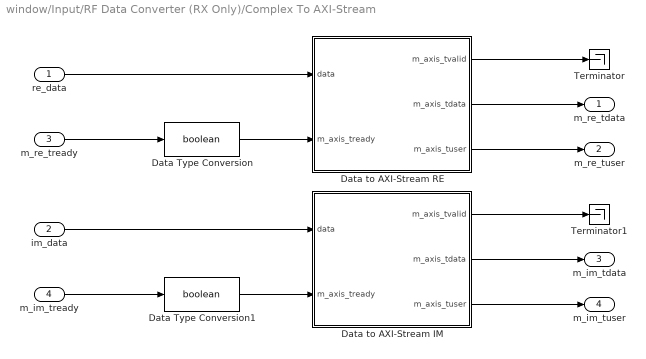
== system window/Input/RF Data Converter (RX Only)/Complex To AXI-Stream ==
  re_data : Inport
  im_data : Inport  Port=2
  m_re_tready : Inport  Port=3
  m_im_tready : Inport  Port=4
  Data Type Conversion : DataTypeConversion  OutDataTypeStr=boolean
  Data Type Conversion1 : DataTypeConversion  OutDataTypeStr=boolean
  Data to AXI-Stream IM : Subsystem
  Data to AXI-Stream RE : Subsystem
  Terminator : Terminator
  Terminator1 : Terminator
  m_re_tdata : Outport  VectorParamsAs1DForOutWhenUnconnected=off
  m_re_tuser : Outport  Port=2  VectorParamsAs1DForOutWhenUnconnected=off
  m_im_tdata : Outport  Port=3  VectorParamsAs1DForOutWhenUnconnected=off
  m_im_tuser : Outport  Port=4  VectorParamsAs1DForOutWhenUnconnected=off
  wires:
  Data Type Conversion1/1 -> Data to AXI-Stream IM/2(m_axis_tready)
  Data Type Conversion/1 -> Data to AXI-Stream RE/2(m_axis_tready)
  re_data/1 -> Data to AXI-Stream RE/1(data)
  m_im_tready/1 -> Data Type Conversion1/1
  Data to AXI-Stream RE/2(m_axis_tdata) -> m_re_tdata/1
  m_re_tready/1 -> Data Type Conversion/1
  Data to AXI-Stream RE/1(m_axis_tvalid) -> Terminator/1
  Data to AXI-Stream IM/2(m_axis_tdata) -> m_im_tdata/1
  Data to AXI-Stream IM/3(m_axis_tuser) -> m_im_tuser/1
  im_data/1 -> Data to AXI-Stream IM/1(data)
  Data to AXI-Stream RE/3(m_axis_tuser) -> m_re_tuser/1
  Data to AXI-Stream IM/1(m_axis_tvalid) -> Terminator1/1

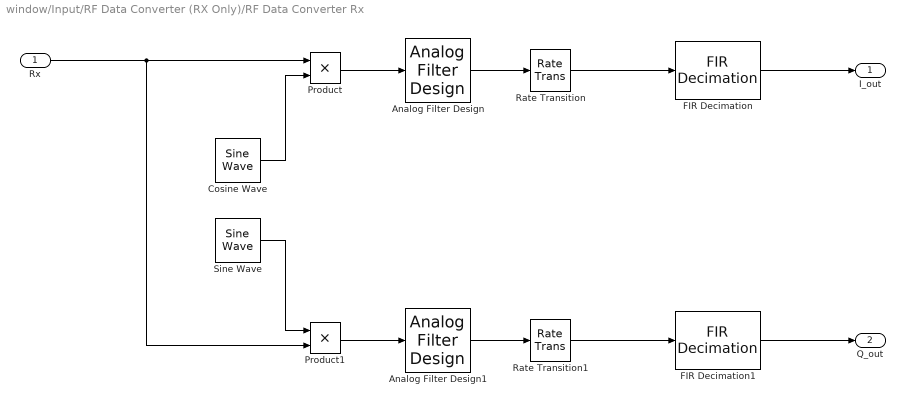
== system window/Input/RF Data Converter (RX Only)/RF Data Converter Rx ==
  Rx : Inport
  Analog Filter Design : dsparch4/Analog Filter Design  method=Butterworth  filttype=Lowpass  N=8  Wlo=2*pi*128e6  Whi=80  Rp=2  Rs=40
  Analog Filter Design1 : dsparch4/Analog Filter Design  method=Butterworth  filttype=Lowpass  N=8  Wlo=2*pi*128e6  Whi=80  Rp=2  Rs=40
  Cosine Wave : dspsrcs4/Sine Wave  Amplitude=1  Frequency=fc_rx  Phase=pi/2  SampleMode=Continuous  OutComplex=Real  CompMethod=Trigonometric fcn  TableSize=Speed  SampleTime=0  SamplesPerFrame=1  ResetState=Restart at time zero  OutputFrames=off  dataType=double  wordLen=16  udDataType=sfix(16)  fracBitsMode=Best precision  numFracBits=15  OutDataTypeStr=double  LastOutDataTypeStr=double
  FIR Decimation : dspmlti4/FIR Decimation  FilterSource=Auto  h=designMultirateFIR(1,2)  D=4  filtStruct=Direct form  FilterObject=FDECIM  framing=Enforce single-rate processing  inputOffset=0  outputBufInitCond=0  roundingMode=Floor  overflowMode=off  firstCoeffDataTypeStr=Inherit: Same word length as input  firstCoeffMin=[]  firstCoeffMax=[]  firstCoeffLastDataTypeStr=Inherit: Same word length as input  outputDataTypeStr=Inherit: Same as accumulator  outputMin=[]  outputMax=[]  outputLastDataTypeStr=Inherit: Same as accumulator
  FIR Decimation1 : dspmlti4/FIR Decimation  FilterSource=Auto  h=designMultirateFIR(1,2)  D=4  filtStruct=Direct form  FilterObject=FDECIM  framing=Enforce single-rate processing  inputOffset=0  outputBufInitCond=0  roundingMode=Floor  overflowMode=off  firstCoeffDataTypeStr=Inherit: Same word length as input  firstCoeffMin=[]  firstCoeffMax=[]  firstCoeffLastDataTypeStr=Inherit: Same word length as input  outputDataTypeStr=Inherit: Same as accumulator  outputMin=[]  outputMax=[]  outputLastDataTypeStr=Inherit: Same as accumulator
  Product : Product
  Product1 : Product
  Rate Transition : RateTransition  OutPortSampleTime=1/fs
  Rate Transition1 : RateTransition  OutPortSampleTime=1/fs
  Sine Wave : dspsrcs4/Sine Wave  Amplitude=1  Frequency=fc_rx  Phase=pi  SampleMode=Continuous  OutComplex=Real  CompMethod=Trigonometric fcn  TableSize=Speed  SampleTime=1/f  SamplesPerFrame=1  ResetState=Restart at time zero  OutputFrames=off  dataType=double  wordLen=16  udDataType=sfix(16)  fracBitsMode=Best precision  numFracBits=15  OutDataTypeStr=double  LastOutDataTypeStr=double
  I_out : Outport  VectorParamsAs1DForOutWhenUnconnected=off
  Q_out : Outport  Port=2  VectorParamsAs1DForOutWhenUnconnected=off
  wires:
  Analog Filter Design1/1 -> Rate Transition1/1
  Analog Filter Design/1 -> Rate Transition/1
  Product1/1 -> Analog Filter Design1/1
  Product/1 -> Analog Filter Design/1
  Rate Transition/1 -> FIR Decimation/1
  FIR Decimation/1 -> I_out/1
  Rate Transition1/1 -> FIR Decimation1/1
  Rx/1 -> Product1/2, Product/1
  Cosine Wave/1 -> Product/2
  Sine Wave/1 -> Product1/1
  FIR Decimation1/1 -> Q_out/1

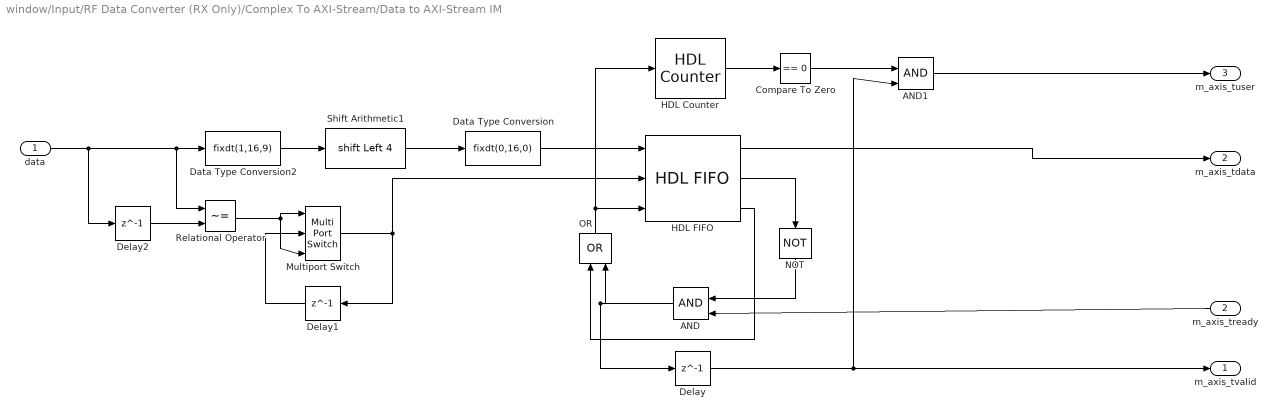
== system window/Input/RF Data Converter (RX Only)/Complex To AXI-Stream/Data to AXI-Stream IM ==
  data : Inport
  m_axis_tready : Inport  Port=2
  AND : Logic  IconShape=distinctive  AllPortsSameDT=off  OutDataTypeStr=boolean
  AND1 : Logic  IconShape=distinctive  AllPortsSameDT=off  OutDataTypeStr=boolean
  Compare To Zero : simulink/Logic and Bit Operations/Compare To Zero  relop===  OutDataTypeStr=boolean
  Data Type Conversion : DataTypeConversion  OutDataTypeStr=fixdt(0,16,0)  ConvertRealWorld=Stored Integer (SI)
  Data Type Conversion2 : DataTypeConversion  OutDataTypeStr=fixdt(1,16,9)
  Delay : Delay  DelayLength=1
  Delay1 : Delay  DelayLength=1
  Delay2 : Delay  DelayLength=1
  HDL Counter : hdlsllib/Sources/HDL Counter  CountType=Count limited  CountInit=0  CountStep=1  CountMax=2^11-1  CountFromType=Initial value  CountFrom=0  CountResetPort=off  CountLoadPort=off  CountEnbPort=on  CountDirPort=off  CountDataType=Unsigned  CountWordLen=32  CountFracLen=0  CountSampTime=1
  HDL FIFO : hdlsllib/HDL RAMs/HDL FIFO  fifo_size=256  mode=Classic  ratio=1  push_msg=Error  pop_msg=Error  show_empty=on  show_full=on  show_num=off  LabelModeActiveChoice_Mode=Classic
      settings: SourceProductBaseCode=SL
  Multiport Switch : MultiPortSwitch  DataPortOrder=Zero-based contiguous  Inputs=2  zeroidx=on
  NOT : Logic  Operator=NOT  IconShape=distinctive  AllPortsSameDT=off  OutDataTypeStr=boolean
  OR : Logic  Operator=OR  IconShape=distinctive  AllPortsSameDT=off  OutDataTypeStr=boolean
  Relational Operator : RelationalOperator  Operator=~=  OutDataTypeStr=boolean  RndMeth=Simplest
  Shift Arithmetic1 : ArithShift  BitShiftNumber=4  BitShiftDirection=Left
  m_axis_tvalid : Outport  VectorParamsAs1DForOutWhenUnconnected=off
  m_axis_tdata : Outport  Port=2  VectorParamsAs1DForOutWhenUnconnected=off
  m_axis_tuser : Outport  Port=3  VectorParamsAs1DForOutWhenUnconnected=off
  wires:
  HDL FIFO/1 -> m_axis_tdata/1
  AND1/1 -> m_axis_tuser/1
  Compare To Zero/1 -> AND1/1
  HDL Counter/1 -> Compare To Zero/1
  HDL FIFO/2 -> NOT/1
  Delay/1 -> AND1/2, m_axis_tvalid/1
  NOT/1 -> AND/1
  m_axis_tready/1 -> AND/2
  data/1 -> Delay2/1, Relational Operator/1, Data Type Conversion2/1
  Multiport Switch/1 -> HDL FIFO/2, Delay1/1
  Delay1/1 -> Multiport Switch/2
  Relational Operator/1 -> Multiport Switch/3, Multiport Switch/1
  Delay2/1 -> Relational Operator/2
  AND/1 -> Delay/1, OR/2
  HDL FIFO/3 -> OR/1
  OR/1 -> HDL FIFO/3, HDL Counter/1
  Data Type Conversion2/1 -> Shift Arithmetic1/1
  Shift Arithmetic1/1 -> Data Type Conversion/1
  Data Type Conversion/1 -> HDL FIFO/1

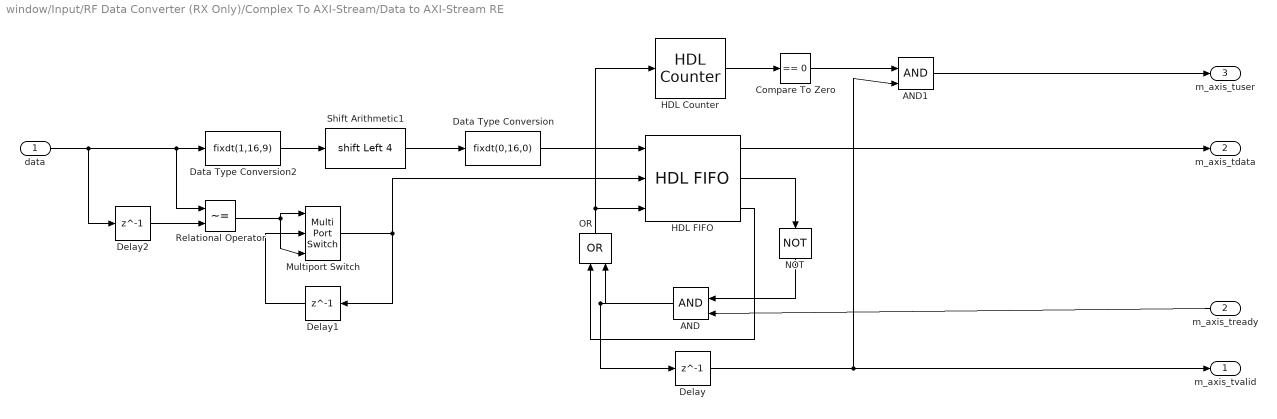
== system window/Input/RF Data Converter (RX Only)/Complex To AXI-Stream/Data to AXI-Stream RE ==
  data : Inport
  m_axis_tready : Inport  Port=2
  AND : Logic  IconShape=distinctive  AllPortsSameDT=off  OutDataTypeStr=boolean
  AND1 : Logic  IconShape=distinctive  AllPortsSameDT=off  OutDataTypeStr=boolean
  Compare To Zero : simulink/Logic and Bit Operations/Compare To Zero  relop===  OutDataTypeStr=boolean
  Data Type Conversion : DataTypeConversion  OutDataTypeStr=fixdt(0,16,0)  ConvertRealWorld=Stored Integer (SI)
  Data Type Conversion2 : DataTypeConversion  OutDataTypeStr=fixdt(1,16,9)
  Delay : Delay  DelayLength=1
  Delay1 : Delay  DelayLength=1
  Delay2 : Delay  DelayLength=1
  HDL Counter : hdlsllib/Sources/HDL Counter  CountType=Count limited  CountInit=0  CountStep=1  CountMax=2^11-1  CountFromType=Initial value  CountFrom=0  CountResetPort=off  CountLoadPort=off  CountEnbPort=on  CountDirPort=off  CountDataType=Unsigned  CountWordLen=32  CountFracLen=0  CountSampTime=1
  HDL FIFO : hdlsllib/HDL RAMs/HDL FIFO  fifo_size=256  mode=Classic  ratio=1  push_msg=Error  pop_msg=Error  show_empty=on  show_full=on  show_num=off  LabelModeActiveChoice_Mode=Classic
      settings: SourceProductBaseCode=SL
  Multiport Switch : MultiPortSwitch  DataPortOrder=Zero-based contiguous  Inputs=2  zeroidx=on
  NOT : Logic  Operator=NOT  IconShape=distinctive  AllPortsSameDT=off  OutDataTypeStr=boolean
  OR : Logic  Operator=OR  IconShape=distinctive  AllPortsSameDT=off  OutDataTypeStr=boolean
  Relational Operator : RelationalOperator  Operator=~=  OutDataTypeStr=boolean  RndMeth=Simplest
  Shift Arithmetic1 : ArithShift  BitShiftNumber=4  BitShiftDirection=Left
  m_axis_tvalid : Outport  VectorParamsAs1DForOutWhenUnconnected=off
  m_axis_tdata : Outport  Port=2  VectorParamsAs1DForOutWhenUnconnected=off
  m_axis_tuser : Outport  Port=3  VectorParamsAs1DForOutWhenUnconnected=off
  wires:
  Data Type Conversion/1 -> HDL FIFO/1
  Shift Arithmetic1/1 -> Data Type Conversion/1
  Data Type Conversion2/1 -> Shift Arithmetic1/1
  OR/1 -> HDL Counter/1, HDL FIFO/3
  HDL FIFO/3 -> OR/1
  AND/1 -> OR/2, Delay/1
  Delay2/1 -> Relational Operator/2
  Relational Operator/1 -> Multiport Switch/1, Multiport Switch/3
  Delay1/1 -> Multiport Switch/2
  Multiport Switch/1 -> Delay1/1, HDL FIFO/2
  data/1 -> Data Type Conversion2/1, Relational Operator/1, Delay2/1
  m_axis_tready/1 -> AND/2
  NOT/1 -> AND/1
  Delay/1 -> m_axis_tvalid/1, AND1/2
  HDL FIFO/2 -> NOT/1
  HDL Counter/1 -> Compare To Zero/1
  Compare To Zero/1 -> AND1/1
  AND1/1 -> m_axis_tuser/1
  HDL FIFO/1 -> m_axis_tdata/1

== matlab function window/Input/Window Generation ==
  data: en output; window_length input; coeff_out output; window_type input
% Generates the window types. Stepping through the windows with larger step
% sizes gives smaller window lengths. This is because when generating the
% windows, the length parameter has to be constant. 
%
% Case 4 is the IDLE state and will only change to another state if either
% the window length or type has been changed in the mask. 

function [en,coeff_out] = fcn(window_length,window_type)

persistent count state prev_param 

if isempty(count)
    count = 0;
    state = 5;
    prev_param = [99 99];
end

window_max = 2048;

hamming_coeffs = hamming(window_max);
hann_coeffs = hann(window_max);
blackman_coeffs = blackman(window_max);
rectangular_coeffs = rectwin(window_max);
debug_coeffs = (1:2048)/2048;

step = window_max/window_length;

switch state
    case 0 
        if count < window_max
            count = count + step;
            coeff_out = hamming_coeffs(count);
            en = true;
        else
            en = false;
            state = 5;
            coeff_out = 0;
        end

    case 1
        if count < window_max
            count = count + step;
            coeff_out = hann_coeffs(count);
            en = true;
        else
            en = false;
            state = 5;
            coeff_out = 0;
        end
        
    case 2   
        if count < window_max
            count = count + step;
            coeff_out = blackman_coeffs(count);
            en = true;
        else
            en = false;
            state = 5;
            coeff_out = 0;
        end
        
    case 3   
        if count < window_max
            count = count + step;
            coeff_out = rectangular_coeffs(count);
            en = true;
        else
            en = false;
            state = 5;
            coeff_out = 0;
        end
        
    case 4
        if count < window_max
            count = count + step;
            coeff_out = debug_coeffs(count);
            en = true;
        else
            en = false;
            state = 5;
            coeff_out = 0;
        end
        
    case 5
        count = 0;
        en = false;
        coeff_out = 0;
        curr_param = [window_type window_length];
        
        if any(curr_param(:) ~= prev_param(:))
            state = window_type;
            prev_param = [window_type window_length];
        end
        
    otherwise
        coeff_out = 0;
        state = 5;
        en = false;
end

== matlab function window/Input/MATLAB Function ==
  data: en input; y output; factor input
function y = fcn(en, factor)

persistent count

if isempty(count)
    count = 0;
end

if en   
    count = count + 1;
    if count >= factor
        y = true;
        count = 0;
    else
        y = false;
    end
else
    y = false;
end

== matlab function window/Reconfigurable Window/MATLAB Function1 ==
  data: d_count input; fifo_read output; w_count input; address output; window_load output; data_valid output; data_tlast output; data_tuser output; window_size parameter; debug output
function [fifo_read, address, window_load, data_valid, data_tlast, data_tuser, debug] = window_fsm(d_count, w_count,window_size)
% Define FSM States
WAIT = 0;
WINDOW_LOAD = 1;
FRAME_START = 2;
READ_FIFO = 3;
FRAME_END = 4;
POPULATE = 5;

size = window_size - 1;

persistent state addr window_loaded

if isempty(state)
    state = fi(0,0,3,0);
    addr = fi(0,0,log2(window_size),0);
    window_loaded = false;
end

switch state
        
    case WAIT
        % Set outputs
        fifo_read = true;
        address = addr;
        window_load = false;
        data_valid = false;
        data_tlast = false;
        data_tuser = fi(0,0,1,0);
        debug = state;
        
        if w_count >= size
            addr(:) = 0;
            state(:) = WINDOW_LOAD;
        elseif d_count >= size && addr == 0
            state(:) = FRAME_START;
        elseif window_loaded && d_count < size
            state(:) = POPULATE;
        end
        
    case WINDOW_LOAD
        % Set outputs
        fifo_read = true;
        address = addr;
        window_load = true;
        data_valid = false;
        data_tlast = false;
        data_tuser = fi(0,0,1,0);
        debug = state;
        
        addr(:) = addr + 1;
            
        if addr >= size && d_count >= size
            window_loaded = true;
            state(:) = FRAME_START;
            addr(:) = 0;
        elseif addr >= size && d_count < size
            window_loaded = true;
            state(:) = WAIT;
            addr(:) = 0;
        end
        
        
    case FRAME_START
        % Set outputs
        fifo_read = true;
        address = addr;
        window_load = false;
        data_valid = true;
        data_tlast = false;
        data_tuser = fi(1,0,1,0);
        debug = state;
        
        addr(:) = addr + 1;
        
        state(:) = READ_FIFO;
            
    case READ_FIFO
        % Set outputs       
        fifo_read = true;
        address = addr;
        window_load = false;
        data_valid = true;
        data_tlast = false;
        data_tuser = fi(0,0,1,0);
        debug = state;
          
        addr(:) = addr + 1;
            
        if addr >= size
            state(:) = FRAME_END;
        end

    case FRAME_END
        % Set outputs       
        fifo_read = true;
        address = addr;
        window_load = false;
        data_valid = true;
        data_tlast = true;
        data_tuser = fi(0,0,1,0);
        debug = state;
        
        addr(:) = 0;
        
        if w_count >= size
            state(:) = WINDOW_LOAD;
        elseif d_count < size
            state(:) = WAIT;
        else
            state(:) = FRAME_START;
        end
        
    case POPULATE
        fifo_read = false;
        address = addr;
        window_load = false;
        data_valid = false;
        data_tlast = false;
        data_tuser = fi(0,0,1,0);
        debug = state;
        
        if d_count >= size
            state(:) = FRAME_START;
        end
        
    otherwise
        % Set outputs
        fifo_read = false;
        address = addr;
        window_load = false;
        data_valid = false;
        data_tlast = false;
        data_tuser = fi(0,0,1,0);
        debug = state;
        
        % Reset variables
        addr(:) = 0;
        
        state(:) = WAIT;
        
end
